simulink model "EGRVlv_VDSens"  (R2018a)
settings: configuration reference "cs_ert" (kept outside this file)
model workspace (MAT data in the model file):
  EGRVlv_VDSens_DT = 10
values from neighbouring files (symbols this model uses):
  EGRVlv_facPT1_C = 50.0    [EGRVlv_VDSens.sldd]
  EGRVlv_facPT1ModVal_C = 50.0    [EGRVlv_VDSens.sldd]
  EGRVlv_rActMax_C = 95.0    [EGRVlv_VDSens.sldd]
  EGRVlv_rActMin_C = 5.0    [EGRVlv_VDSens.sldd]
  EGRVlv_rActOfs_C = 0.0    [EGRVlv_VDSens.sldd]
  EGRVlv_rCmpNewCtlUn_C = 20.0    [EGRVlv_VDSens.sldd]
  EGRVlv_RmpSlpNeg_C = 3.0    [EGRVlv_VDSens.sldd]
  EGRVlv_RmpSlpPos_C = 3.0    [EGRVlv_VDSens.sldd]
  EGRVlv_rPullDwnThres_C = 15.0    [EGRVlv_VDSens.sldd]
  EGRVlv_rTmpOfsLrnMax_C = 30.0    [EGRVlv_VDSens.sldd]
  EGRVlv_rTmpOfsLrnMin_C = 10.0    [EGRVlv_VDSens.sldd]
  EGRVlv_rTransStgDfl_C = 20.0    [EGRVlv_VDSens.sldd]
  EGRVlv_swtActOfs_C = 0.0    [EGRVlv_VDSens.sldd]
  EGRVlv_swtOfsLrnActv_C = 1.0    [EGRVlv_VDSens.sldd]
  EGRVlv_swtSensPrs_C = 1.0    [EGRVlv_VDSens.sldd]
  SigTst_rEGRVlv_C = 20.0    [EGRVlv_VDSens.sldd]
  SigTst_swtEGRVlv_C = 0    [EGRVlv_VDSens.sldd]
undefined symbols (not defined in the file or in its folder): CEngDst_switch_conv, Switch
libraries: sllib x3, simulink x2
settings Model: DataDictionary=EGRVlv_VDSens.sldd  Creator=zhoutinglin  LastModifiedBy=zhoutinglin

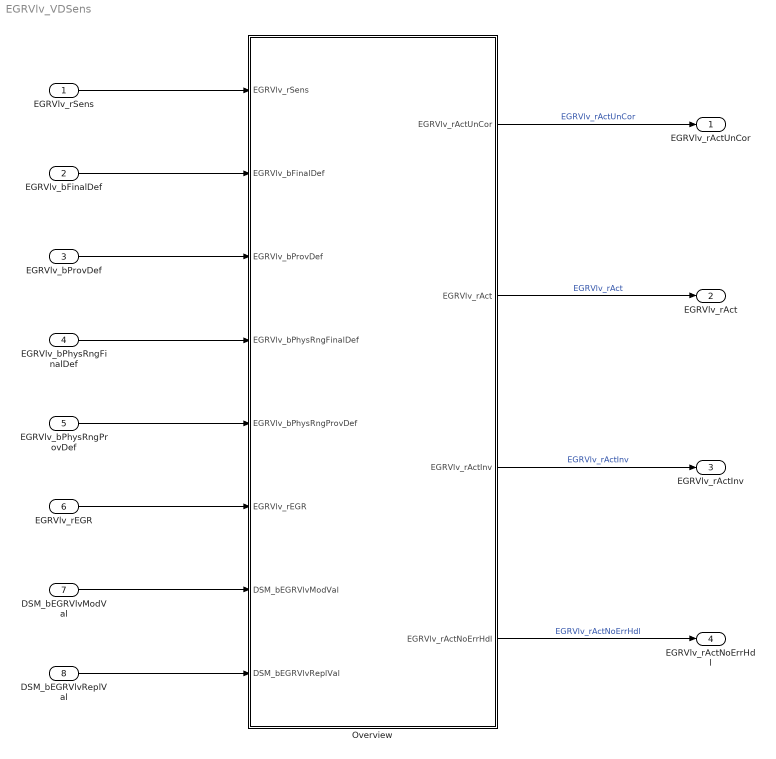
== system EGRVlv_VDSens ==
  EGRVlv_rSens : Inport  Description=Sensed value of actuator position without error handling  OutMin=-100  OutMax=100  OutDataTypeStr=DutyCycle  Unit=%  PortDimensions=[1 1]
  EGRVlv_bFinalDef : Inport  Description=the final fault flag  Port=2  OutMin=0  OutMax=1  OutDataTypeStr=boolean  PortDimensions=[1 1]
  EGRVlv_bProvDef : Inport  Description=the fault flag for the moment  Port=3  OutMin=0  OutMax=1  OutDataTypeStr=boolean  PortDimensions=[1 1]
  EGRVlv_bPhysRngFinalDef : Inport  Description=Status Sensor of the EGR valve physical Signal range check finally defect  Port=4  OutMin=0  OutMax=1  OutDataTypeStr=boolean  PortDimensions=[1 1]
  EGRVlv_bPhysRngProvDef : Inport  Description=Status Sensor of the EGR valve physical Signal range check temporary defect  Port=5  OutMin=0  OutMax=1  OutDataTypeStr=boolean  PortDimensions=[1 1]
  EGRVlv_rEGR : Inport  Description=Control value for the EGR valve  Port=6  OutMin=-100  OutMax=100  OutDataTypeStr=DutyCycle  Unit=%  PortDimensions=[1 1]
  DSM_bEGRVlvModVal : Inport  Description=Status of FId_EGRVlvModVal  Port=7  OutMin=0  OutMax=1  OutDataTypeStr=boolean  PortDimensions=[1 1]
  DSM_bEGRVlvReplVal : Inport  Description=Desired value from LMS control  Port=8  OutMin=0  OutMax=1  OutDataTypeStr=boolean  PortDimensions=[1 1]
  Overview : Subsystem
  EGRVlv_rActUnCor : Outport
  EGRVlv_rAct : Outport  Port=2
  EGRVlv_rActInv : Outport  Port=3
  EGRVlv_rActNoErrHdl : Outport  Port=4
  wires:
  EGRVlv_bPhysRngFinalDef/1 -> Overview/4(EGRVlv_bPhysRngFinalDef)
  EGRVlv_rSens/1 -> Overview/1(EGRVlv_rSens)
  EGRVlv_bFinalDef/1 -> Overview/2(EGRVlv_bFinalDef)
  EGRVlv_bProvDef/1 -> Overview/3(EGRVlv_bProvDef)
  EGRVlv_bPhysRngProvDef/1 -> Overview/5(EGRVlv_bPhysRngProvDef)
  EGRVlv_rEGR/1 -> Overview/6(EGRVlv_rEGR)
  DSM_bEGRVlvModVal/1 -> Overview/7(DSM_bEGRVlvModVal)
  DSM_bEGRVlvReplVal/1 -> Overview/8(DSM_bEGRVlvReplVal)
  Overview/1(EGRVlv_rActUnCor) -> EGRVlv_rActUnCor/1  "EGRVlv_rActUnCor"
  Overview/2(EGRVlv_rAct) -> EGRVlv_rAct/1  "EGRVlv_rAct"
  Overview/3(EGRVlv_rActInv) -> EGRVlv_rActInv/1  "EGRVlv_rActInv"
  Overview/4(EGRVlv_rActNoErrHdl) -> EGRVlv_rActNoErrHdl/1  "EGRVlv_rActNoErrHdl"

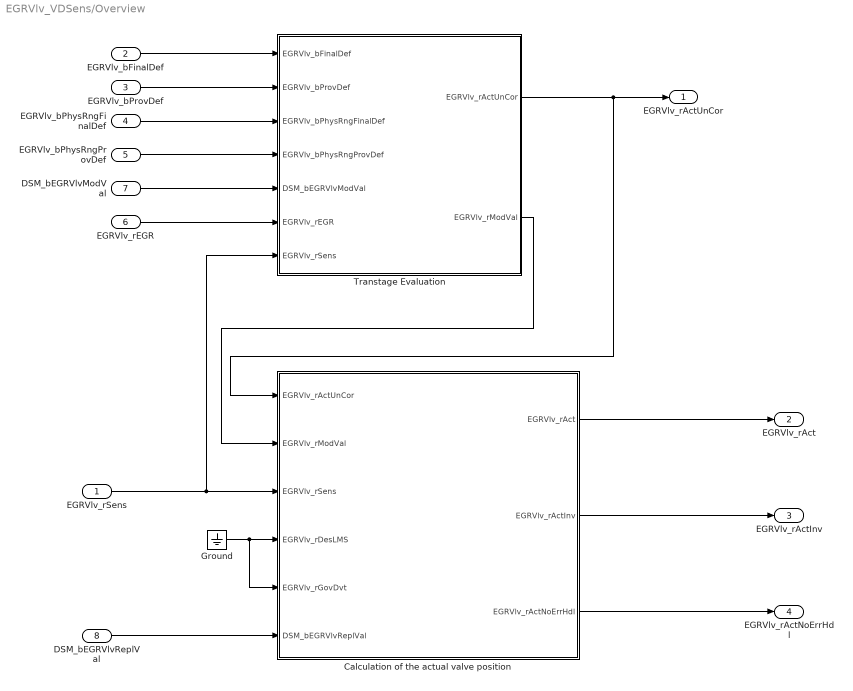
== system EGRVlv_VDSens/Overview ==
  EGRVlv_rSens : Inport  Tag=%
  EGRVlv_bFinalDef : Inport  Port=2
  EGRVlv_bProvDef : Inport  Port=3
  EGRVlv_bPhysRngFinalDef : Inport  Port=4
  EGRVlv_bPhysRngProvDef : Inport  Port=5
  EGRVlv_rEGR : Inport  Tag=%  Port=6
  DSM_bEGRVlvModVal : Inport  Tag=%  Port=7
  DSM_bEGRVlvReplVal : Inport  Tag=%  Port=8
  Calculation of the actual valve position : Subsystem
  Ground : Ground
  Transtage Evaluation : Subsystem
  EGRVlv_rActUnCor : Outport  Tag=%
  EGRVlv_rAct : Outport  Tag=%  Port=2
  EGRVlv_rActInv : Outport  Tag=%  Port=3
  EGRVlv_rActNoErrHdl : Outport  Port=4
  wires:
  Transtage Evaluation/1(EGRVlv_rActUnCor) -> Calculation of the actual valve position/1(EGRVlv_rActUnCor), EGRVlv_rActUnCor/1
  EGRVlv_rSens/1 -> Transtage Evaluation/7(EGRVlv_rSens), Calculation of the actual valve position/3(EGRVlv_rSens)
  EGRVlv_rEGR/1 -> Transtage Evaluation/6(EGRVlv_rEGR)
  EGRVlv_bFinalDef/1 -> Transtage Evaluation/1(EGRVlv_bFinalDef)
  EGRVlv_bProvDef/1 -> Transtage Evaluation/2(EGRVlv_bProvDef)
  EGRVlv_bPhysRngFinalDef/1 -> Transtage Evaluation/3(EGRVlv_bPhysRngFinalDef)
  EGRVlv_bPhysRngProvDef/1 -> Transtage Evaluation/4(EGRVlv_bPhysRngProvDef)
  DSM_bEGRVlvModVal/1 -> Transtage Evaluation/5(DSM_bEGRVlvModVal)
  Ground/1 -> Calculation of the actual valve position/5(EGRVlv_rGovDvt), Calculation of the actual valve position/4(EGRVlv_rDesLMS)
  DSM_bEGRVlvReplVal/1 -> Calculation of the actual valve position/6(DSM_bEGRVlvReplVal)
  Calculation of the actual valve position/1(EGRVlv_rAct) -> EGRVlv_rAct/1
  Calculation of the actual valve position/2(EGRVlv_rActInv) -> EGRVlv_rActInv/1
  Calculation of the actual valve position/3(EGRVlv_rActNoErrHdl) -> EGRVlv_rActNoErrHdl/1
  Transtage Evaluation/2(EGRVlv_rModVal) -> Calculation of the actual valve position/2(EGRVlv_rModVal)

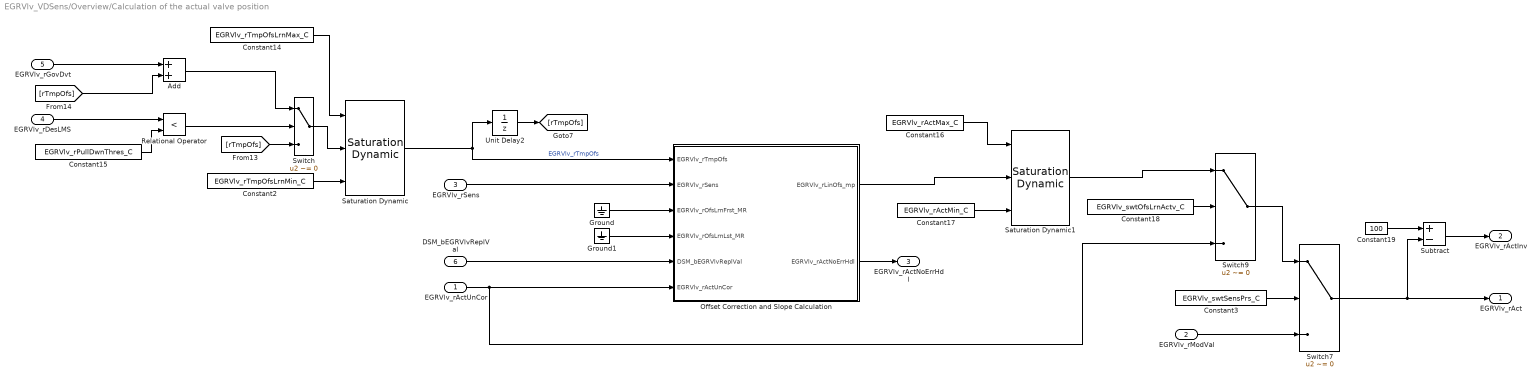
== system EGRVlv_VDSens/Overview/Calculation of the actual valve position ==
  EGRVlv_rActUnCor : Inport  Tag=%
  EGRVlv_rModVal : Inport  Tag=%  Port=2
  EGRVlv_rSens : Inport  Tag=%  Port=3
  EGRVlv_rDesLMS : Inport  Port=4
  EGRVlv_rGovDvt : Inport  Port=5
  DSM_bEGRVlvReplVal : Inport  Tag=%  Port=6
  Add : Sum  SaturateOnIntegerOverflow=on
  Constant14 : Constant  Value=EGRVlv_rTmpOfsLrnMax_C  SampleTime=-1
  Constant15 : Constant  Value=EGRVlv_rPullDwnThres_C  SampleTime=-1
  Constant16 : Constant  Value=EGRVlv_rActMax_C  SampleTime=-1
  Constant17 : Constant  Value=EGRVlv_rActMin_C  SampleTime=-1
  Constant18 : Constant  Value=EGRVlv_swtOfsLrnActv_C  SampleTime=-1
  Constant19 : Constant  Value=100  OutDataTypeStr=Inherit: Inherit via back propagation
  Constant2 : Constant  Value=EGRVlv_rTmpOfsLrnMin_C  SampleTime=-1
  Constant3 : Constant  Value=EGRVlv_swtSensPrs_C
  Ground : Ground
  Ground1 : Ground
  Offset Correction and Slope Calculation : Subsystem
  Relational Operator : RelationalOperator  Operator=<  OutDataTypeStr=boolean  RndMeth=Simplest
  Saturation Dynamic : simulink/Discontinuities/Saturation Dynamic  OutMin=[]  OutMax=[]  OutDataTypeStr=Inherit: Same as second input  OutDataType=fixdt(1, 16)  OutScaling=2^-10  DoSatur=off
  Saturation Dynamic1 : simulink/Discontinuities/Saturation Dynamic  OutMin=[]  OutMax=[]  OutDataTypeStr=Inherit: Same as second input  OutDataType=fixdt(1, 16)  OutScaling=2^-10  DoSatur=off
  Subtract : Sum  Inputs=+-  SaturateOnIntegerOverflow=on  InputSameDT=on
  Switch : Switch  Criteria=u2 ~= 0
  Switch7 : Switch  Criteria=u2 ~= 0  Threshold=CEngDst_switch_conv.OFF  InputSameDT=on
  Switch9 : Switch  Criteria=u2 ~= 0  Threshold=CEngDst_switch_conv.OFF  InputSameDT=on
  Unit Delay2 : UnitDelay  SampleTime=-1
      settings: AttributesFormatString=InitialValue=%<InitialCondition>
  EGRVlv_rAct : Outport  Tag=%
  EGRVlv_rActInv : Outport  Tag=%  Port=2
  EGRVlv_rActNoErrHdl : Outport  Port=3
  wires:
  Constant3/1 -> Switch7/2
  Switch7/1 -> EGRVlv_rAct/1, Subtract/2
  Constant14/1 -> Saturation Dynamic/1
  Constant2/1 -> Saturation Dynamic/3
  Constant15/1 -> Relational Operator/2
  EGRVlv_rDesLMS/1 -> Relational Operator/1
  Relational Operator/1 -> Switch/2
  EGRVlv_rGovDvt/1 -> Add/1
  Add/1 -> Switch/1
  [rTmpOfs] -> Switch/3
  Switch/1 -> Saturation Dynamic/2
  Saturation Dynamic/1 -> Offset Correction and Slope Calculation/1(EGRVlv_rTmpOfs), Unit Delay2/1  "EGRVlv_rTmpOfs"
  [rTmpOfs] -> Add/2
  Constant16/1 -> Saturation Dynamic1/1
  Saturation Dynamic1/1 -> Switch9/1
  Constant18/1 -> Switch9/2
  Constant17/1 -> Saturation Dynamic1/3
  Switch9/1 -> Switch7/1
  Offset Correction and Slope Calculation/1(EGRVlv_rLinOfs_mp) -> Saturation Dynamic1/2
  Constant19/1 -> Subtract/1
  Subtract/1 -> EGRVlv_rActInv/1
  Unit Delay2/1 -> [rTmpOfs]
  EGRVlv_rModVal/1 -> Switch7/3
  EGRVlv_rActUnCor/1 -> Offset Correction and Slope Calculation/6(EGRVlv_rActUnCor), Switch9/3
  EGRVlv_rSens/1 -> Offset Correction and Slope Calculation/2(EGRVlv_rSens)
  DSM_bEGRVlvReplVal/1 -> Offset Correction and Slope Calculation/5(DSM_bEGRVlvReplVal)
  Offset Correction and Slope Calculation/2(EGRVlv_rActNoErrHdl) -> EGRVlv_rActNoErrHdl/1
  Ground1/1 -> Offset Correction and Slope Calculation/4(EGRVlv_rOfsLrnLst_MR)
  Ground/1 -> Offset Correction and Slope Calculation/3(EGRVlv_rOfsLrnFrst_MR)

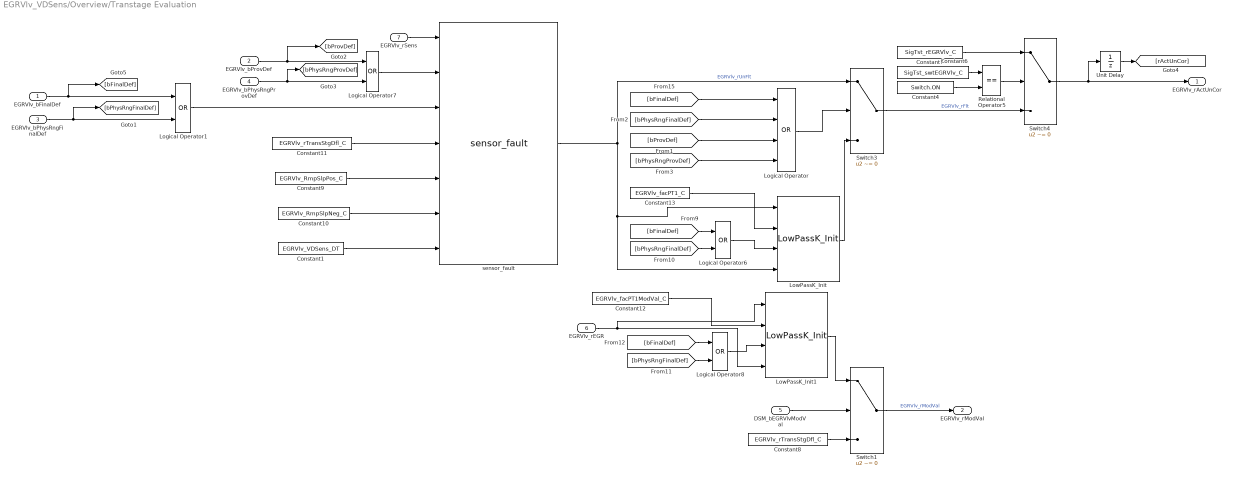
== system EGRVlv_VDSens/Overview/Transtage Evaluation ==
  EGRVlv_bFinalDef : Inport
  EGRVlv_bProvDef : Inport  Port=2
  EGRVlv_bPhysRngFinalDef : Inport  Port=3
  EGRVlv_bPhysRngProvDef : Inport  Port=4
  DSM_bEGRVlvModVal : Inport  Tag=%  Port=5
  EGRVlv_rEGR : Inport  Tag=%  Port=6
  EGRVlv_rSens : Inport  Tag=%  Port=7
  Constant1 : Constant  Value=EGRVlv_VDSens_DT  OutDataTypeStr=Inherit: Inherit via back propagation
  Constant10 : Constant  Value=EGRVlv_RmpSlpNeg_C  SampleTime=-1
  Constant11 : Constant  Value=EGRVlv_rTransStgDfl_C  SampleTime=-1
  Constant12 : Constant  Value=EGRVlv_facPT1ModVal_C
  Constant13 : Constant  Value=EGRVlv_facPT1_C  SampleTime=-1
  Constant4 : Constant  Value=Switch.ON
  Constant6 : Constant  Value=SigTst_swtEGRVlv_C  SampleTime=-1
  Constant7 : Constant  Value=SigTst_rEGRVlv_C  SampleTime=-1
  Constant8 : Constant  Value=EGRVlv_rTransStgDfl_C
  Constant9 : Constant  Value=EGRVlv_RmpSlpPos_C  SampleTime=-1
  Logical Operator : Logic  Operator=OR  Inputs=4  OutDataTypeStr=boolean
  Logical Operator{1,6..8} (4 alike) : Logic  Operator=OR  OutDataTypeStr=boolean
  LowPassK_Init : sllib/LowPassK_Init
      settings: SourceProductName=sllib
  LowPassK_Init1 : sllib/LowPassK_Init
      settings: SourceProductName=sllib
  Relational Operator5 : RelationalOperator  Operator===  OutDataTypeStr=boolean  RndMeth=Simplest  InputSameDT=on
  Switch1 : Switch  Criteria=u2 ~= 0  Threshold=CEngDst_switch_conv.OFF  InputSameDT=on
  Switch3 : Switch  Criteria=u2 ~= 0  InputSameDT=on
  Switch4 : Switch  Criteria=u2 ~= 0  Threshold=CEngDst_switch_conv.OFF  InputSameDT=on
  Unit Delay : UnitDelay  SampleTime=-1
      settings: AttributesFormatString=InitialValue=%<InitialCondition>
  sensor_fault : sllib/sensor_fault
      settings: SourceProductName=sllib
  EGRVlv_rActUnCor : Outport  Tag=%
  EGRVlv_rModVal : Outport  Tag=%  Port=2
  wires:
  Constant6/1 -> Relational Operator5/1
  Logical Operator1/1 -> sensor_fault/3
  Relational Operator5/1 -> Switch4/2
  [bPhysRngProvDef] -> Logical Operator/4
  [bPhysRngFinalDef] -> Logical Operator6/2
  [bFinalDef] -> Logical Operator6/1
  Constant4/1 -> Relational Operator5/2
  [bProvDef] -> Logical Operator/3
  [bPhysRngFinalDef] -> Logical Operator/2
  Logical Operator6/1 -> LowPassK_Init/3
  Constant1/1 -> sensor_fault/7
  LowPassK_Init/1 -> Switch3/3
  Constant9/1 -> sensor_fault/5
  EGRVlv_bPhysRngProvDef/1 -> Logical Operator7/2, [bPhysRngProvDef]
  Logical Operator7/1 -> sensor_fault/2
  Constant7/1 -> Switch4/1
  [bFinalDef] -> Logical Operator/1
  Unit Delay/1 -> [rActUnCor]
  EGRVlv_bFinalDef/1 -> Logical Operator1/1, [bFinalDef]
  Constant10/1 -> sensor_fault/6
  EGRVlv_bPhysRngFinalDef/1 -> Logical Operator1/2, [bPhysRngFinalDef]
  Constant13/1 -> LowPassK_Init/2
  EGRVlv_bProvDef/1 -> Logical Operator7/1, [bProvDef]
  Logical Operator/1 -> Switch3/2
  EGRVlv_rSens/1 -> sensor_fault/1
  sensor_fault/1 -> Switch3/1, LowPassK_Init/4, LowPassK_Init/1  "EGRVlv_rUnFlt"
  Switch3/1 -> Switch4/3  "EGRVlv_rFlt"
  Switch4/1 -> Unit Delay/1, EGRVlv_rActUnCor/1
  DSM_bEGRVlvModVal/1 -> Switch1/2
  Switch1/1 -> EGRVlv_rModVal/1  "EGRVlv_rModVal"
  Constant8/1 -> Switch1/3
  LowPassK_Init1/1 -> Switch1/1
  EGRVlv_rEGR/1 -> LowPassK_Init1/4, LowPassK_Init1/1
  Constant12/1 -> LowPassK_Init1/2
  [bPhysRngFinalDef] -> Logical Operator8/2
  [bFinalDef] -> Logical Operator8/1
  Logical Operator8/1 -> LowPassK_Init1/3
  Constant11/1 -> sensor_fault/4

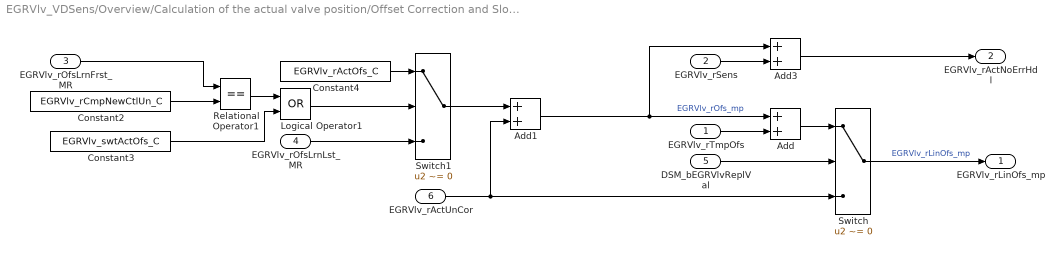
== system EGRVlv_VDSens/Overview/Calculation of the actual valve position/Offset Correction and Slope Calculation ==
  EGRVlv_rTmpOfs : Inport  Tag=%
  EGRVlv_rSens : Inport  Tag=%  Port=2
  EGRVlv_rOfsLrnFrst_MR : Inport  Tag=%  Port=3
  EGRVlv_rOfsLrnLst_MR : Inport  Tag=%  Port=4
  DSM_bEGRVlvReplVal : Inport  Tag=%  Port=5
  EGRVlv_rActUnCor : Inport  Tag=%  Port=6
  Add : Sum  SaturateOnIntegerOverflow=on
  Add1 : Sum  SaturateOnIntegerOverflow=on
  Add3 : Sum  SaturateOnIntegerOverflow=on
  Constant2 : Constant  Value=EGRVlv_rCmpNewCtlUn_C  SampleTime=-1
  Constant3 : Constant  Value=EGRVlv_swtActOfs_C  SampleTime=-1
  Constant4 : Constant  Value=EGRVlv_rActOfs_C  SampleTime=-1
  Logical Operator1 : Logic  Operator=OR  AllPortsSameDT=off  OutDataTypeStr=boolean
  Relational Operator1 : RelationalOperator  Operator===  OutDataTypeStr=boolean  RndMeth=Simplest
  Switch : Switch  Criteria=u2 ~= 0
  Switch1 : Switch  Criteria=u2 ~= 0
  EGRVlv_rLinOfs_mp : Outport
  EGRVlv_rActNoErrHdl : Outport  Port=2
  wires:
  EGRVlv_rSens/1 -> Add3/2
  EGRVlv_rTmpOfs/1 -> Add/2
  Switch/1 -> EGRVlv_rLinOfs_mp/1  "EGRVlv_rLinOfs_mp"
  Add3/1 -> EGRVlv_rActNoErrHdl/1
  DSM_bEGRVlvReplVal/1 -> Switch/2
  Constant2/1 -> Relational Operator1/2
  EGRVlv_rOfsLrnFrst_MR/1 -> Relational Operator1/1
  Relational Operator1/1 -> Logical Operator1/1
  Constant3/1 -> Logical Operator1/2
  Logical Operator1/1 -> Switch1/2
  EGRVlv_rOfsLrnLst_MR/1 -> Switch1/3
  Constant4/1 -> Switch1/1
  Add1/1 -> Add/1, Add3/1  "EGRVlv_rOfs_mp"
  Add/1 -> Switch/1
  Switch1/1 -> Add1/1
  EGRVlv_rActUnCor/1 -> Add1/2, Switch/3
